simulink model "part1_q7"  (R2023b)
settings: Solver=VariableStepAuto  StartTime=0.0  StopTime=100  RelTol=1e-3
values from neighbouring files (symbols this model uses):
  A = 1.2    [part1_q4.m]
  Cd = 0.5    [part1_q4.m]
  f = 0.015    [part1_q4.m]    (also in th4_q19.m; th4_q19_claude.m)
  g = 9.81    [part1_q4.m]    (also in th4_q19.m; th4_q19_claude.m; th4_q19_create_road_grade.m = segments(i,3))
  m = 1250    [part1_q4.m]    (also in th4_q19_battery_pps.m = 1305.3)
  m_eqv = m + I_w_total/r^2 + I_e*(G*R)^2/r^2    (= 1305.28194444)    [part1_q4.m]    (also in th4_q19.m = 1305.3; th4_q19_claude.m = 1305.3)
  ro = 1.225    [part1_q4.m]
  theta_0 = 0    [part1_q4.m]
  u_w = 2    [part1_q4.m]
libraries: simulink_extras x1, slpidlib x1
settings Model: Creator=yusufcagriogut  LastModifiedBy=yusufcagriogut

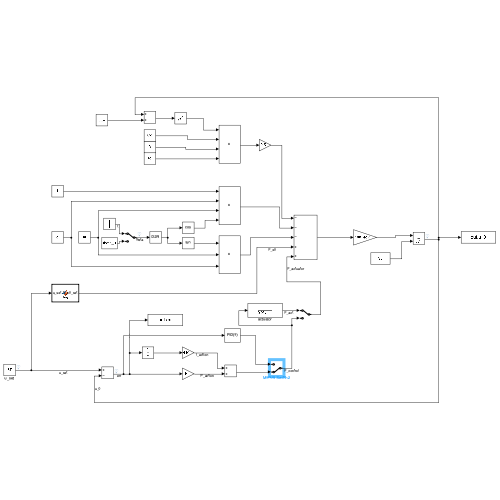
[thumbnail: Simulink's stored preview of the top-level diagram]
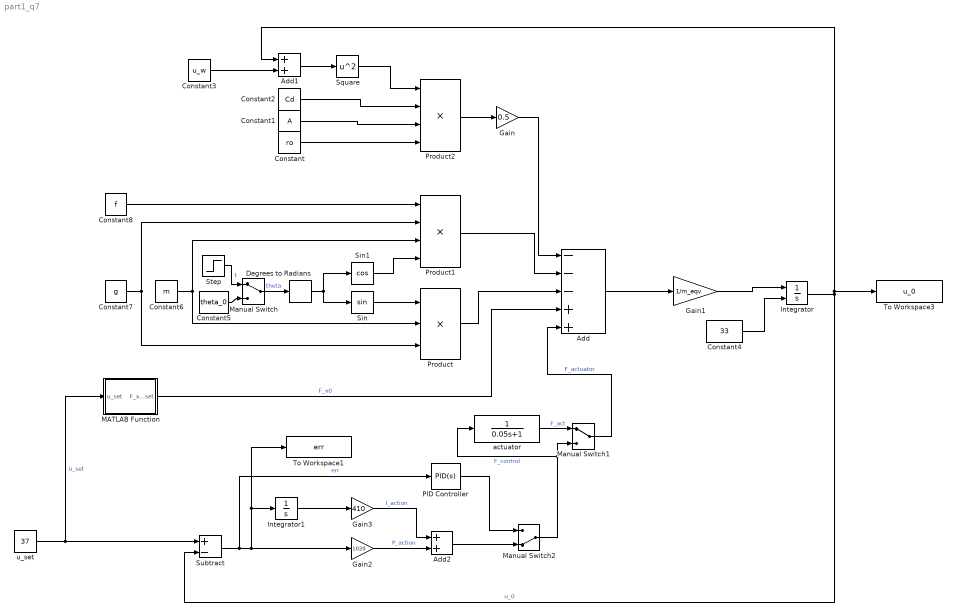
== system part1_q7 ==
  Add : Sum  Inputs=---++
  Add1 : Sum
  Add2 : Sum
  Constant : Constant  Value=ro
  Constant1 : Constant  Value=A
  Constant2 : Constant  Value=Cd
  Constant3 : Constant  Value=u_w
  Constant4 : Constant  Value=33
  Constant5 : Constant  Value=theta_0
  Constant6 : Constant  Value=m
  Constant7 : Constant  Value=g
  Constant8 : Constant  Value=f
  Degrees to Radians : simulink_extras/Transformations/Degrees to Radians
  Gain : Gain  Gain=0.5
  Gain1 : Gain  Gain=1/m_eqv
  Gain2 : Gain  Gain=1020
  Gain3 : Gain  Gain=410
  Integrator : Integrator  InitialConditionSource=external  InitialCondition=33
  Integrator1 : Integrator
  MATLAB Function : MATLAB Function  TreatAsAtomicUnit=on
  Manual Switch : ManualSwitch
  Manual Switch1 : ManualSwitch
  Manual Switch2 : ManualSwitch  CurrentSetting=0
  PID Controller : slpidlib/PID Controller  Controller=PID  Form=Parallel  TimeDomain=Continuous-time  UseExternalTs=off  SampleTime=-1  IntegratorMethod=Forward Euler  FilterMethod=Forward Euler  ControllerParametersSource=internal  P=2916.18008245389  I=1185.46038349683  UseKiTs=off  D=369.124172057518  N=12.815158437423  UseFilter=on  TunerSelectOption=Transfer Function Based (PID Tuner App)  InitialConditionSource=internal  InitialConditionForIntegrator=0  InitialConditionForFilter=0  DifferentiatorICPrevScaledInput=0  ExternalReset=none  TrackingMode=off  Kt=1  LimitOutput=off  SatLimitsSource=internal  UpperSaturationLimit=inf  LowerSaturationLimit=-inf  LinearizeAsGain=on  AntiWindupMode=none  Kb=1  LimitIntegrator=off  UpperIntegratorSaturationLimit=inf  LowerIntegratorSaturationLimit=-inf  POutMin=[]  POutMax=[]  IOutMin=[]  IOutMax=[]  DOutMin=[]  DOutMax=[]  NOutMin=[]  NOutMax=[]  SumOutMin=[]  SumOutMax=[]  SaturationOutMin=[]  SaturationOutMax=[]  PParamMin=[]  PParamMax=[]  IParamMin=[]  IParamMax=[]  DParamMin=[]  DParamMax=[]  NParamMin=[]  NParamMax=[]  KbParamMin=[]  KbParamMax=[]  KtParamMin=[]  KtParamMax=[]  KbOutMin=[]  KbOutMax=[]  KtOutMin=[]  KtOutMax=[]  IntegratorOutMin=[]  IntegratorOutMax=[]  FilterOutMin=[]  FilterOutMax=[]  SumI1OutMin=[]  SumI1OutMax=[]  SumI2OutMin=[]  SumI2OutMax=[]  SumI3OutMin=[]  SumI3OutMax=[]  SumI4OutMin=[]  SumI4OutMax=[]  SumDOutMin=[]  SumDOutMax=[]  DifferentiatorOutMin=[]  DifferentiatorOutMax=[]  FilterDiffOutCoefMin=[]  FilterDiffOutCoefMax=[]  ReciprocalOutMin=[]  ReciprocalOutMax=[]  SumDenOutMin=[]  SumDenOutMax=[]  SumNumOutMin=[]  SumNumOutMax=[]  DivideOutMin=[]  DivideOutMax=[]  UdiffTsProdOutMin=[]  UdiffTsProdOutMax=[]  NTsProdOutMin=[]  NTsProdOutMax=[]  UintegralTsProdOutMin=[]  UintegralTsProdOutMax=[]  UngainTsProdOutMin=[]  UngainTsProdOutMax=[]  ClampingZeroOutDataTypeStr=Inherit: Inherit via back propagation  ClampingZeroOutMin=[]  ClampingZeroOutMax=[]  FilterDenConstantOutDataTypeStr=Inherit: Inherit via back propagation  FilterDenConstantOutMin=[]  FilterDenConstantOutMax=[]  PCopyOutDataTypeStr=Inherit: Inherit via back propagation  PCopyOutMin=[]  PCopyOutMax=[]  NCopyOutDataTypeStr=Inherit: Inherit via back propagation  NCopyOutMin=[]  NCopyOutMax=[]  IntegratorContinuousStateAttributes=''  IntegratorStateMustResolveToSignalObject=off  IntegratorRTWStateStorageClass=Auto  FilterContinuousStateAttributes=''  FilterStateMustResolveToSignalObject=off  FilterRTWStateStorageClass=Auto  ParallelPVariant=InternalParameters  IdealPVariant=Disabled  IVariant=InternalParameters  DVariant=InternalParameters  IntegratorVariant=Continuous  SatVariant=Disabled  AWVariant=Passthrough  PCopyVariant=Disabled  TRVariant=Disabled  FdbkBlocksVariant=Forward  IdealPFdbkVariant=Disabled  SatFdbkVariant=Disabled  DerivativeFilterVariant=ContFilter  NVariant=InternalParameters  NCopyVariant=Disabled  FilterICVariant=InternalICsFilter  IntegratorICVariant=InternalICs  ExternalResetVariant=Disabled  TRSumVariant=Passthrough  SumFdbkVariant=Disabled  SumVariant=Sum_PID  TsampFilterVariant=InternalTs  TsampNgainVariant=Passthrough  TsampIntegralVariant=Disabled_SignalSpec  ExternalSaturationOutDataTypeStr=Inherit: Same as second input
  Product : Product  Inputs=3
  Product1 : Product  Inputs=4
  Product2 : Product  Inputs=4
  Sin : Trigonometry
  Sin1 : Trigonometry  Operator=cos
  Square : Math  Operator=square
  Step : Step  Time=0  Before=7  After=7  SampleTime=0
  Subtract : Sum  Inputs=+-
  To Workspace1 : ToWorkspace  VariableName=err  SaveFormat=Timeseries  SampleTime=-1
  To Workspace3 : ToWorkspace  VariableName=u_0  SaveFormat=Timeseries  SampleTime=-1
  actuator : TransferFcn  Denominator=[0.05 1]
  u_set : Constant  Value=37
  wires:
  Sin/1 -> Product/1
  Constant7/1 -> Product/3, Product1/2
  Product/1 -> Add/3
  Sin1/1 -> Product1/4
  Constant6/1 -> Product/2, Product1/3
  Constant8/1 -> Product1/1
  Product1/1 -> Add/2
  Product2/1 -> Gain/1
  Gain/1 -> Add/1
  Constant/1 -> Product2/4
  Constant1/1 -> Product2/3
  Constant2/1 -> Product2/2
  Add1/1 -> Square/1
  Constant3/1 -> Add1/2
  Add/1 -> Gain1/1
  Gain1/1 -> Integrator/1
  Integrator/1 -> To Workspace3/1, Add1/1, Subtract/2  "u_0"
  u_set/1 -> MATLAB Function/1(u_set), Subtract/1  "u_set"
  Subtract/1 -> PID Controller/1, To Workspace1/1, Integrator1/1, Gain2/1  "err"
  Integrator1/1 -> Gain3/1
  Gain2/1 -> Add2/2  "P_action"
  Gain3/1 -> Add2/1  "I_action"
  MATLAB Function/1(F_x0_set) -> Add/4  "F_x0"
  Square/1 -> Product2/1
  Constant4/1 -> Integrator/2
  Degrees to Radians/1 -> Sin/1, Sin1/1
  Manual Switch/1 -> Degrees to Radians/1  "theta"
  Step/1 -> Manual Switch/1  "t"
  Constant5/1 -> Manual Switch/2
  actuator/1 -> Manual Switch1/1  "F_act"
  Manual Switch1/1 -> Add/5  "F_actuator"
  Add2/1 -> Manual Switch2/2
  PID Controller/1 -> Manual Switch2/1
  Manual Switch2/1 -> Manual Switch1/2, actuator/1  "F_control"

== matlab function part1_q7/MATLAB Function ==
  data: u_set input; F_x0_set output
function F_x0_set = fcn(u_set)
m = 1250;
ro = 1.225;
A = 1.2;
Cd = 0.5;
f = 0.015;
R = 3;
I_e = 0.15;
r = 0.3;
I_w = 1.0;
u_0 = 40;
u_w = 2;
g = 9.81;
theta_0 = 0;
F_x0_set = m*g*sin(theta_0) + f*m*g*cos(theta_0) + ...
    0.5*ro*A*Cd*(u_set+u_w)^2;
end
